simulink model "IM_Global_Control"  (R2021a)
settings: Solver=FixedStepDiscrete  StartTime=0.0  StopTime=10.0  FixedStep=1e-5  RelTol=1e-3
undefined symbols (not defined in the file): DiscIntNeverNeededParam, sigbuilder_block
libraries: simulink x4
settings Model: Creator=Mehra  LastModifiedBy=Mehra

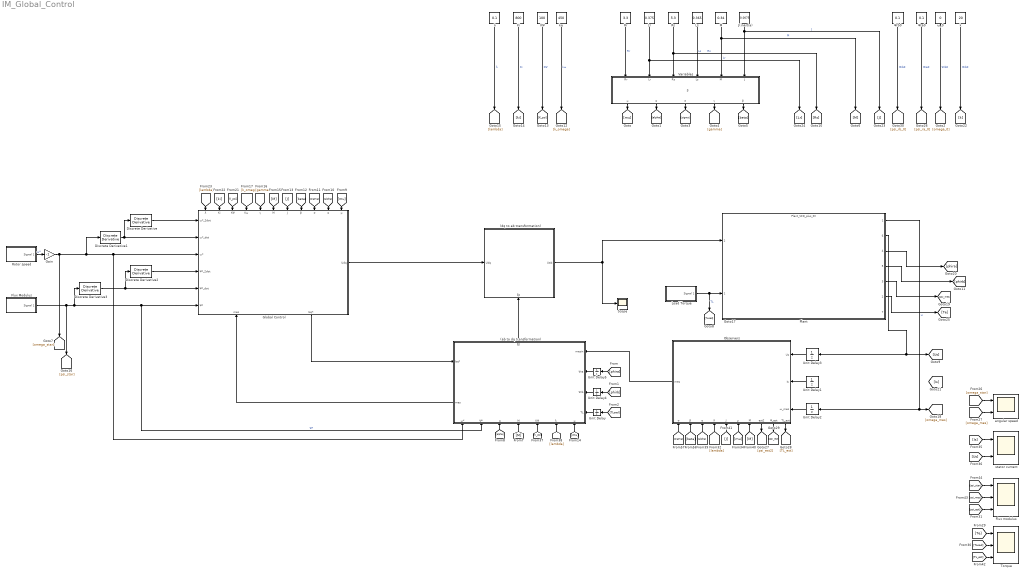
== system IM_Global_Control ==
  note: β
  (ab to dq transformation) : Subsystem
      settings: PortSchema="{\"entries\":[{\"content\":{\"sides\":[{\"content\":{\"connectorIds\":[\"In1\",\"Out2\"]},\"type\":\"ConnectorPlacement.EquallySpacedRectSide\",\"uuid\":\"954ddc6c-32ec-4fca-997a-51b3ced09e6e\"},{\"content\":{\"connectorIds\":[\"In9\",\"In10\",\"In11\",\"In12\"],\"side\":\"RIGHT\"},\"type\":\"ConnectorPlacement.EquallySpacedRectSide\",\"uuid\":\"d23f0106-fd66-41c5-9167-f0bfa2e5f0d7\"},{\"content\":{\"connectorIds\":[\"Out1\"],\"side\":\"TOP\"},\"type\":\"ConnectorPlacement.EquallySpacedRectSide\",\"uuid\":\"ec2ab734-74ce-4c08-89a8-e0d0cab377a3\"},{\"content\":{\"connectorIds\":[\"In2\",\"In3\",\"In4\",\"In5\",\"In6\",\"In7\",\"In8\"],\"side\":\"BOTTOM\"},\"type\":\"ConnectorPlacement.EquallySpacedRectSide\",\"uuid\":\"e8fbabf1-c1e7-4b41-8038-4f25f2d2c141\"}]},\"type\":\"ConnectorPlacement.EquallySpacedConnector\",\"uuid\":\"2eb72d65-4150-4441-ba17-035a64db8a78\"}],\"packageUris\":[\"http://schema.mathworks.com/mf0/Connector/R2020b\"],\"version\":\"1.0\"}"
  (dq to ab transformation) : Subsystem
      settings: PortSchema="{\"entries\":[{\"content\":{\"sides\":[{\"content\":{\"connectorIds\":[\"In1\"]},\"type\":\"ConnectorPlacement.EquallySpacedRectSide\",\"uuid\":\"fcc9e9c0-f3ff-45b3-b4d9-89988d9b9a34\"},{\"content\":{\"connectorIds\":[\"Out1\"],\"side\":\"RIGHT\"},\"type\":\"ConnectorPlacement.EquallySpacedRectSide\",\"uuid\":\"b8117d1c-eda8-48ca-a376-b80f3451eb1b\"},{\"content\":{\"connectorIds\":[],\"side\":\"TOP\"},\"type\":\"ConnectorPlacement.EquallySpacedRectSide\",\"uuid\":\"632a2e27-4ebf-4489-a7a1-4102ed33f7de\"},{\"content\":{\"connectorIds\":[\"In2\"],\"side\":\"BOTTOM\"},\"type\":\"ConnectorPlacement.EquallySpacedRectSide\",\"uuid\":\"b1ed2b98-7899-49a7-98d1-ff7a05505f88\"}]},\"type\":\"ConnectorPlacement.EquallySpacedConnector\",\"uuid\":\"0e689d41-d128-44ad-a484-465e7f7df4f8\"}],\"packageUris\":[\"http://schema.mathworks.com/mf0/Connector/R2020b\"],\"version\":\"1.0\"}"
  Discrete Derivative{,1..3} (4 alike) : simulink/Discrete/Discrete Derivative  gainval=1.0  ICPrevScaledInput=0.0  OutMin=[]  OutMax=[]  OutDataType=fixdt(1, 16)  OutScaling=2^-10  DoSatur=off
  Flux Modulus : Subsystem  Tag=STV Subsys  LoadFcn=sigbuilder_block('load');  StartFcn=sigbuilder_block('start');  StopFcn=sigbuilder_block('stop');  ClipboardFcn=sigbuilder_block('clipboard');  mask(Sigbuilder block){tuvar=[0:10]}
      mask help: Simulink:masks:SigbuilderBlock_MD
      mask init:
      | if ~strcmp(get_param(bdroot(gcbh),'SimulationStatus'),'stopped') tuvar = sigbuilder_block('maskInit'); end
      settings: CopyFcn=sigbuilder_block('copy');  DeleteFcn=sigbuilder_block('delete');  ModelCloseFcn=sigbuilder_block('modelClose');  PreSaveFcn=sigbuilder_block('preSave');  PauseFcn=sigbuilder_block('pause');  ContinueFcn=sigbuilder_block('continue');  NameChangeFcn=sigbuilder_block('namechange');  OpenFcn=sigbuilder_block('open',[433.8 177.6 550.8 400.2 ]);  CloseFcn=sigbuilder_block('close');
      mask Display: plot(0, 0, 100, 100,[2, 2, 32, 32, 2], [68, 8, 8, 68, 68],[32, 2], [38, 38], [32, 19, 2],[53, 60, 44], [32, 17, 17, 2],[16, 16, 31, 31]);txt = getActiveGroup(gcbh);text(2, 100, txt,'verticalAlignment', 'top');
  Flux modulus : Scope  NumInputPorts=3
  Gain : Gain  Gain=-1
  Global Control : Subsystem
      settings: PortSchema="{\"entries\":[{\"content\":{\"sides\":[{\"content\":{\"connectorIds\":[\"In1\",\"In2\",\"In3\",\"In4\",\"In5\",\"In6\"]},\"type\":\"ConnectorPlacement.EquallySpacedRectSide\",\"uuid\":\"d7ac22ed-73dc-4923-8a02-de2b77bc4b56\"},{\"content\":{\"connectorIds\":[\"Out1\"],\"side\":\"RIGHT\"},\"type\":\"ConnectorPlacement.EquallySpacedRectSide\",\"uuid\":\"0ed82d2d-ac01-4440-b414-7b739c3193d9\"},{\"content\":{\"connectorIds\":[\"In7\",\"In8\",\"In9\",\"In10\",\"In11\",\"In12\",\"In13\",\"In14\",\"In15\",\"In16\",\"In17\"],\"side\":\"TOP\"},\"type\":\"ConnectorPlacement.EquallySpacedRectSide\",\"uuid\":\"be3374af-951c-49b1-9762-82694f1e2186\"},{\"content\":{\"connectorIds\":[\"In18\",\"Out2\"],\"side\":\"BOTTOM\"},\"type\":\"ConnectorPlacement.EquallySpacedRectSide\",\"uuid\":\"0e0cdf13-df45-4d83-96ab-036d988b30e8\"}]},\"type\":\"ConnectorPlacement.EquallySpacedConnector\",\"uuid\":\"01640f11-0e41-43e3-9a6d-1e07964cb7e3\"}],\"packageUris\":[\"http://schema.mathworks.com/mf0/Connector/R2020b\"],\"version\":\"1.0\"}"
  J(inertia) : Constant  Value=0.0075
  Ki : Constant  Value=800
  KΨ : Constant  Value=100
  Load Torque : Subsystem  Tag=STV Subsys  LoadFcn=sigbuilder_block('load');  StartFcn=sigbuilder_block('start');  StopFcn=sigbuilder_block('stop');  ClipboardFcn=sigbuilder_block('clipboard');  mask(Sigbuilder block){tuvar=[0:10]}
      mask help: Simulink:masks:SigbuilderBlock_MD
      mask init:
      | if ~strcmp(get_param(bdroot(gcbh),'SimulationStatus'),'stopped') tuvar = sigbuilder_block('maskInit'); end
      settings: CopyFcn=sigbuilder_block('copy');  DeleteFcn=sigbuilder_block('delete');  ModelCloseFcn=sigbuilder_block('modelClose');  PreSaveFcn=sigbuilder_block('preSave');  PauseFcn=sigbuilder_block('pause');  ContinueFcn=sigbuilder_block('continue');  NameChangeFcn=sigbuilder_block('namechange');  OpenFcn=sigbuilder_block('open',[418.2 149.4 550.8 400.2 ]);  CloseFcn=sigbuilder_block('close');
      mask Display: plot(0, 0, 100, 100,[2, 2, 32, 32, 2], [68, 8, 8, 68, 68],[32, 2], [38, 38], [32, 19, 2],[53, 60, 44], [32, 17, 17, 2],[16, 16, 31, 31]);txt = getActiveGroup(gcbh);text(2, 100, txt,'verticalAlignment', 'top');
  Lr : Constant  Value=0.375
  Ls : Constant  Value=0.365
  M : Constant  Value=0.34
  Observers : Subsystem
      settings: PortSchema="{\"entries\":[{\"content\":{\"sides\":[{\"content\":{\"connectorIds\":[\"In1\",\"In2\",\"In3\"]},\"type\":\"ConnectorPlacement.EquallySpacedRectSide\",\"uuid\":\"a75d3ae5-6cbc-4a81-a14c-a9660c01f407\"},{\"content\":{\"connectorIds\":[\"Out1\"],\"side\":\"RIGHT\"},\"type\":\"ConnectorPlacement.EquallySpacedRectSide\",\"uuid\":\"810d57cb-fd51-4174-8429-89dcdd7ccf2e\"},{\"content\":{\"connectorIds\":[],\"side\":\"TOP\"},\"type\":\"ConnectorPlacement.EquallySpacedRectSide\",\"uuid\":\"084f081f-5dfb-4a02-b6e7-31480db1dce2\"},{\"content\":{\"connectorIds\":[\"Out2\",\"Out3\",\"Out4\",\"In4\",\"In5\",\"In6\",\"In7\",\"In8\",\"In9\",\"In10\"],\"side\":\"BOTTOM\"},\"type\":\"ConnectorPlacement.EquallySpacedRectSide\",\"uuid\":\"ad0ec213-e44f-4285-8d86-85a591b1b38d\"}]},\"type\":\"ConnectorPlacement.EquallySpacedConnector\",\"uuid\":\"2b9d98d5-99d7-45ac-aedf-db0f18522aa3\"}],\"packageUris\":[\"http://schema.mathworks.com/mf0/Connector/R2020b\"],\"version\":\"1.0\"}"
  Plant : ModelReference  ModelNameDialog=Plant_VFD_plus_IM.slx  SimulationMode=Normal  ModelReferenceVersion=1.1162
      settings: PortSchema="{\"entries\":[{\"content\":{\"sides\":[{\"content\":{\"connectorIds\":[\"In2\",\"In1\"]},\"type\":\"ConnectorPlacement.EquallySpacedRectSide\",\"uuid\":\"ada58a5e-1472-4b56-9b66-b9d99a7685f5\"},{\"content\":{\"connectorIds\":[\"Out1\",\"Out6\",\"Out4\",\"Out5\",\"Out3\",\"Out2\",\"Out7\"],\"side\":\"RIGHT\"},\"type\":\"ConnectorPlacement.EquallySpacedRectSide\",\"uuid\":\"42b90cbf-75bc-499b-a3c1-3c9b222f35d5\"},{\"content\":{\"connectorIds\":[],\"side\":\"TOP\"},\"type\":\"ConnectorPlacement.EquallySpacedRectSide\",\"uuid\":\"c9789acb-3ca3-4ea3-b872-57f6132d0fb2\"},{\"content\":{\"connectorIds\":[],\"side\":\"BOTTOM\"},\"type\":\"ConnectorPlacement.EquallySpacedRectSide\",\"uuid\":\"000e5c64-e399-41cd-9c94-e7f3b3194d1a\"}]},\"type\":\"ConnectorPlacement.EquallySpacedConnector\",\"uuid\":\"64f9ad12-90f4-47a3-8034-21f20e745ad8\"}],\"packageUris\":[\"http://schema.mathworks.com/mf0/Connector/R2020b\"],\"version\":\"1.0\"}"
  Rotor speed : Subsystem  Tag=STV Subsys  LoadFcn=sigbuilder_block('load');  StartFcn=sigbuilder_block('start');  StopFcn=sigbuilder_block('stop');  ClipboardFcn=sigbuilder_block('clipboard');  mask(Sigbuilder block){tuvar=[0:10]}
      mask help: Simulink:masks:SigbuilderBlock_MD
      mask init:
      | if ~strcmp(get_param(bdroot(gcbh),'SimulationStatus'),'stopped') tuvar = sigbuilder_block('maskInit'); end
      settings: CopyFcn=sigbuilder_block('copy');  DeleteFcn=sigbuilder_block('delete');  ModelCloseFcn=sigbuilder_block('modelClose');  PreSaveFcn=sigbuilder_block('preSave');  PauseFcn=sigbuilder_block('pause');  ContinueFcn=sigbuilder_block('continue');  NameChangeFcn=sigbuilder_block('namechange');  OpenFcn=sigbuilder_block('open',[418.2 149.4 550.8 400.2 ]);  CloseFcn=sigbuilder_block('close');
      mask Display: plot(0, 0, 100, 100,[2, 2, 32, 32, 2], [68, 8, 8, 68, 68],[32, 2], [38, 38], [32, 19, 2],[53, 60, 44], [32, 17, 17, 2],[16, 16, 31, 31]);txt = getActiveGroup(gcbh);text(2, 100, txt,'verticalAlignment', 'top');
  Rr : Constant  Value=3.3
  Rs : Constant  Value=5.3
  Scope : Scope
  Torque : Scope  NumInputPorts=3
  Unit Delay{,1..5} (6 alike) : UnitDelay  SampleTime=-1  HasFrameUpgradeWarning=on
  Variables : Subsystem
  angular speed : Scope  NumInputPorts=2
  k : Constant  Value=20
  kω : Constant  Value=450
  stator current : Scope  NumInputPorts=2
  Ψra0 : Constant  Value=0.1
  Ψrb0 : Constant  Value=0.1
  λ : Constant  Value=0.1
  ω_0 : Constant  Value=0
  wires:
  [sigma] -> Global Control/15(σ)
  [Us] -> stator current/2
  [omega_star] -> angular speed/1
  [ki] -> Global Control/8(Ki)
  [K_psi] -> Global Control/9(KΨ)
  [omega_mes] -> angular speed/2
  Discrete Derivative3/1 -> Discrete Derivative2/1, Global Control/5(Ψ*_dot)
  [alpha] -> (ab to dq transformation)/4(α)
  [lambda] -> Global Control/7(λ)
  [k_omega] -> Global Control/10(Kω)
  Discrete Derivative/1 -> Global Control/1(ω*_2dot)
  [M] -> (ab to dq transformation)/5(M)
  [psi_star] -> Flux modulus/1
  [TLoad] -> Torque/2
  [M] -> Global Control/12(M)
  Observers/3(Ψ_est) -> [psi_est]
  [Te] -> Torque/1
  [Is] -> stator current/1
  [TL_est] -> Torque/3
  Unit Delay2/1 -> Observers/3(ω_mes)
  (ab to dq transformation)/1(ξ0) -> (dq to ab transformation)/2(ξ0)
  Observers/1(mes) -> (ab to dq transformation)/9(mesin)
  Flux Modulus/1(Signal 1) -> Discrete Derivative3/1, Global Control/6(Ψ*), (ab to dq transformation)/3(Ψ*), [psi_star]  "Ψ*"
  Observers/4(est2) -> [psi_est2]
  Discrete Derivative1/1 -> Discrete Derivative/1, Global Control/2(ω*_dot)
  [mu] -> Global Control/17(µ)
  [beta] -> Global Control/14(β)
  (dq to ab transformation)/1(Uab) -> Scope/1, Plant/2
  [sigma] -> Observers/10(σ)
  [beta] -> Observers/9(β)
  [M] -> Observers/4(M)
  [alpha] -> Observers/8(α)
  [lambda] -> Observers/7(λ)
  [psi_est] -> Flux modulus/3
  Observers/2(TL_est) -> [TL_est]
  [mu] -> Observers/5(µ)
  Global Control/1(Udq) -> (dq to ab transformation)/1(Udq)
  [J] -> Global Control/13(J)
  [gamma] -> Global Control/11(γ)
  [alpha] -> Global Control/16(α)
  [K_psi] -> (ab to dq transformation)/6(KΨ)
  (ab to dq transformation)/2(mes) -> Global Control/18(mes)
  Global Control/2(Isq*) -> (ab to dq transformation)/1(Isq*)
  Discrete Derivative2/1 -> Global Control/4(Ψ*_2dot)
  Rotor speed/1(Signal 1) -> Gain/1  "ω*"
  [lambda] -> (ab to dq transformation)/7(λ)
  [mu] -> (ab to dq transformation)/8(µ)
  [J] -> Observers/6(J)
  [psi_mes] -> Flux modulus/2
  Plant/2 -> [Te]
  Load Torque/1(Signal 1) -> [TLoad], Plant/1  "TL"
  Plant/3 -> [psi_mes]
  Plant/1 -> [omega_mes], Unit Delay2/1  "ω"
  ? -> [Is], Unit Delay1/1
  Plant/6 -> Unit Delay3/1, [Us]
  Unit Delay1/1 -> Observers/2(Is)
  Unit Delay3/1 -> Observers/1(Us)
  Gain/1 -> Discrete Derivative1/1, Global Control/3(ω*), (ab to dq transformation)/2(ω*), [omega_star]
  Plant/5 -> [phirb]
  Plant/4 -> [phira]
  [phira] -> Unit Delay5/1
  [phirb] -> Unit Delay4/1
  [TLoad] -> Unit Delay/1
  Unit Delay/1 -> (ab to dq transformation)/12(TL)
  Unit Delay4/1 -> (ab to dq transformation)/11(Ψrb)
  Unit Delay5/1 -> (ab to dq transformation)/10(Ψra)
  Variables/3(σ) -> [sigma]
  k/1 -> [k]  "Ψrb0"
  Rs/1 -> [Rs], Variables/3(Rs)  "Rs"
  M/1 -> [M], Variables/5(M)  "M"
  Ψrb0/1 -> [psi_rb_0]  "Ψrb0"
  Variables/4(γ) -> [gamma]
  Ψra0/1 -> [psi_ra_0]  "Ψra0"
  Ls/1 -> Variables/4(Ls)  "Ls"
  Variables/2(α) -> [alpha]
  Rr/1 -> Variables/1(Rr)  "Rr"
  ω_0/1 -> [omega_0]  "Ψrb0"
  Variables/5(β) -> [beta]
  Lr/1 -> [Lr], Variables/2(Lr)  "Lr"
  Variables/1(µ) -> [mu]
  J(inertia)/1 -> [J], Variables/6(J)  "J"
  KΨ/1 -> [K_psi]  "KΨ"
  λ/1 -> [lambda]  "λ"
  Ki/1 -> [ki]  "Ki"
  kω/1 -> [k_omega]  "kω"

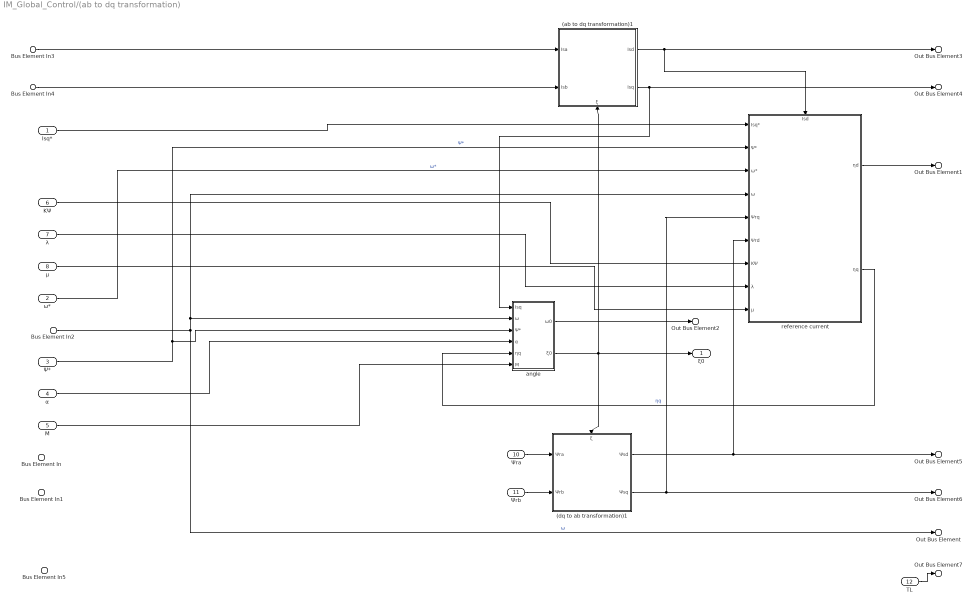
== system IM_Global_Control/(ab to dq transformation) ==
  Isq* : Inport
  ω* : Inport  Port=2
  Ψ* : Inport  Port=3
  α : Inport  Port=4
  M : Inport  Port=5
  KΨ : Inport  Port=6
  λ : Inport  Port=7
  µ : Inport  Port=8
  Bus Element In4 : Inport  Port=9  PortName=mesin  Element=Isb
  Bus Element In : Inport  Port=9  PortName=mesin  Element=Ψra
  Bus Element In1 : Inport  Port=9  PortName=mesin  Element=Ψrb
  Bus Element In2 : Inport  Port=9  PortName=mesin  Element=ω
  Bus Element In3 : Inport  Port=9  PortName=mesin  Element=Isa
  Bus Element In5 : Inport  Port=9  PortName=mesin  Element=TL
  Ψra : Inport  Port=10
  Ψrb : Inport  Port=11
  TL : Inport  Port=12
  (ab to dq transformation)1 : Subsystem
      settings: PortSchema="{\"entries\":[{\"content\":{\"sides\":[{\"content\":{\"connectorIds\":[\"In1\",\"In2\"]},\"type\":\"ConnectorPlacement.EquallySpacedRectSide\",\"uuid\":\"5c330d99-0e0d-44c6-96f8-2a2206da92f9\"},{\"content\":{\"connectorIds\":[\"Out1\",\"Out2\"],\"side\":\"RIGHT\"},\"type\":\"ConnectorPlacement.EquallySpacedRectSide\",\"uuid\":\"d01d6d1d-3c02-43a0-8f85-93fe8d575b38\"},{\"content\":{\"connectorIds\":[],\"side\":\"TOP\"},\"type\":\"ConnectorPlacement.EquallySpacedRectSide\",\"uuid\":\"e1acbeec-a08c-47b9-8afb-d107cbf7174f\"},{\"content\":{\"connectorIds\":[\"In3\"],\"side\":\"BOTTOM\"},\"type\":\"ConnectorPlacement.EquallySpacedRectSide\",\"uuid\":\"e8043408-ca76-4c99-9608-24b05f44ef39\"}]},\"type\":\"ConnectorPlacement.EquallySpacedConnector\",\"uuid\":\"9536c8a8-a5cc-4817-9165-61d2eb9b262d\"}],\"packageUris\":[\"http://schema.mathworks.com/mf0/Connector/R2020b\"],\"version\":\"1.0\"}"
  (dq to ab transformation)1 : Subsystem
      settings: PortSchema="{\"entries\":[{\"content\":{\"sides\":[{\"content\":{\"connectorIds\":[\"In1\",\"In2\"]},\"type\":\"ConnectorPlacement.EquallySpacedRectSide\",\"uuid\":\"5c330d99-0e0d-44c6-96f8-2a2206da92f9\"},{\"content\":{\"connectorIds\":[\"Out1\",\"Out2\"],\"side\":\"RIGHT\"},\"type\":\"ConnectorPlacement.EquallySpacedRectSide\",\"uuid\":\"d01d6d1d-3c02-43a0-8f85-93fe8d575b38\"},{\"content\":{\"connectorIds\":[\"In3\"],\"side\":\"TOP\"},\"type\":\"ConnectorPlacement.EquallySpacedRectSide\",\"uuid\":\"e1acbeec-a08c-47b9-8afb-d107cbf7174f\"},{\"content\":{\"connectorIds\":[],\"side\":\"BOTTOM\"},\"type\":\"ConnectorPlacement.EquallySpacedRectSide\",\"uuid\":\"e8043408-ca76-4c99-9608-24b05f44ef39\"}]},\"type\":\"ConnectorPlacement.EquallySpacedConnector\",\"uuid\":\"9536c8a8-a5cc-4817-9165-61d2eb9b262d\"}],\"packageUris\":[\"http://schema.mathworks.com/mf0/Connector/R2020b\"],\"version\":\"1.0\"}"
  angle : Subsystem
  reference current : Subsystem
      settings: PortSchema="{\"entries\":[{\"content\":{\"sides\":[{\"content\":{\"connectorIds\":[\"In1\",\"In2\",\"In3\",\"In4\",\"In5\",\"In6\",\"In7\",\"In8\",\"In9\"]},\"type\":\"ConnectorPlacement.EquallySpacedRectSide\",\"uuid\":\"20835a9a-3790-4a84-a1cf-3b356ea8ce55\"},{\"content\":{\"connectorIds\":[\"Out1\",\"Out2\"],\"side\":\"RIGHT\"},\"type\":\"ConnectorPlacement.EquallySpacedRectSide\",\"uuid\":\"c7be742b-d8ac-4ccc-8e57-82e64648b197\"},{\"content\":{\"connectorIds\":[\"In10\"],\"side\":\"TOP\"},\"type\":\"ConnectorPlacement.EquallySpacedRectSide\",\"uuid\":\"50541cb9-7339-4b7f-ab09-a0a36464c354\"}]},\"type\":\"ConnectorPlacement.EquallySpacedConnector\",\"uuid\":\"b3e3bb9d-f2d1-405f-a9ca-c5a471d81e39\"}],\"packageUris\":[\"http://schema.mathworks.com/mf0/Connector/R2020b\"],\"version\":\"1.0\"}"
  ξ0 : Outport
  Out Bus Element : Outport  Port=2  PortName=mes  Element=ω
  Out Bus Element1 : Outport  Port=2  PortName=mes  Element=ηd
  Out Bus Element2 : Outport  Port=2  PortName=mes  Element=ω0
  Out Bus Element3 : Outport  Port=2  PortName=mes  Element=Isd
  Out Bus Element4 : Outport  Port=2  PortName=mes  Element=Isq
  Out Bus Element5 : Outport  Port=2  PortName=mes  Element=Ψrd
  Out Bus Element6 : Outport  Port=2  PortName=mes  Element=Ψrq
  Out Bus Element7 : Outport  Port=2  PortName=mes  Element=TL
  wires:
  Ψ*/1 -> angle/3(Ψ*), reference current/2(Ψ*)  "Ψ*"
  Bus Element In2/1 -> Out Bus Element/1, angle/2(ω), reference current/4(ω)  "ω"
  Bus Element In3/1 -> (ab to dq transformation)1/1(Isa)
  Bus Element In4/1 -> (ab to dq transformation)1/2(Isb)
  reference current/2(ηq) -> angle/5(ηq)  "ηq"
  Isq*/1 -> reference current/1(Isq*)
  ω*/1 -> reference current/3(ω*)  "ω*"
  µ/1 -> reference current/9(µ)
  λ/1 -> reference current/8(λ)
  KΨ/1 -> reference current/7(KΨ)
  reference current/1(ηd) -> Out Bus Element1/1
  (ab to dq transformation)1/1(Isd) -> Out Bus Element3/1, reference current/10(Isd)
  (dq to ab transformation)1/1(Ψsd) -> Out Bus Element5/1, reference current/6(Ψrd)
  (dq to ab transformation)1/2(Ψsq) -> Out Bus Element6/1, reference current/5(Ψrq)
  angle/2(ξ0) -> ξ0/1, (dq to ab transformation)1/3(ξ), (ab to dq transformation)1/3(ξ)
  (ab to dq transformation)1/2(Isq) -> angle/1(Isq), Out Bus Element4/1
  α/1 -> angle/4(α)
  M/1 -> angle/6(M)
  angle/1(ω0) -> Out Bus Element2/1
  Ψra/1 -> (dq to ab transformation)1/1(Ψra)
  Ψrb/1 -> (dq to ab transformation)1/2(Ψrb)
  TL/1 -> Out Bus Element7/1

== system IM_Global_Control/(dq to ab transformation) ==
  In Bus Element : Inport  PortName=Udq  Element=usd
  In Bus Element1 : Inport  PortName=Udq  Element=usq
  ξ0 : Inport  Port=2
  Cos : Trigonometry  Operator=cos
  Cos1 : Trigonometry
  Product{,1..3} (4 alike) : Product
  Sin : Trigonometry
  Sin1 : Trigonometry  Operator=cos
  Subtract : Sum  Inputs=+-
  Subtract1 : Sum
  Out Bus Element : Outport  PortName=Uab  Element=Usa
  Out Bus Element1 : Outport  PortName=Uab  Element=Usb
  wires:
  Subtract1/1 -> Out Bus Element1/1  "Usb"
  Subtract/1 -> Out Bus Element/1  "Usa"
  ξ0/1 -> Sin1/1, Cos1/1, Sin/1, Cos/1  "ξ0"
  Cos/1 -> Product/1
  Sin/1 -> Product1/2
  Cos1/1 -> Product2/1
  Sin1/1 -> Product3/2
  In Bus Element/1 -> Product2/2, Product/2  "usd"
  In Bus Element1/1 -> Product3/1, Product1/1  "usq"
  Product/1 -> Subtract/1
  Product1/1 -> Subtract/2
  Product2/1 -> Subtract1/1
  Product3/1 -> Subtract1/2

== system IM_Global_Control/Flux Modulus ==
  Demux : Demux  Tag=STV Demux  Outputs=1
      settings: DisplayOption=none
  FromWs : FromWorkspace  Tag=STV FromWs  VariableName=tuvar
      SigBuilderData=|
      | common.afterFinalStr = 'Extrapolate'
      | common.sampleTime = 0
      | dataSet.timeRange = [0 10]
      | dataSet.name = 'Group 1'
      | sbobj.Groups.Name = 'Group 1'
      | sbobj.Groups.Signals.Name = 'Signal 1'
      | sbobj.Groups.Signals.XData = [0 0.32 1.5 1.8 10]
      | sbobj.Groups.Signals.YData = [0.001 1.16 1.16 0.5 0.5]
  Signal 1 : Outport  Tag=STV Outport
  wires:
  Demux/1 -> Signal 1/1
  FromWs/1 -> Demux/1

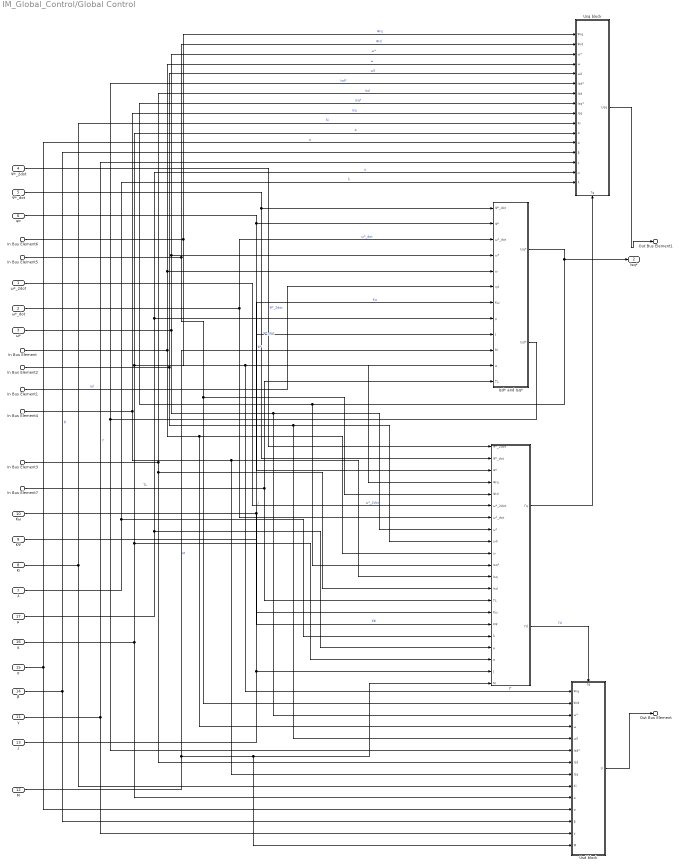
== system IM_Global_Control/Global Control ==
  ω*_2dot : Inport
  ω*_dot : Inport  Port=2
  ω* : Inport  Port=3
  Ψ*_2dot : Inport  Port=4
  Ψ*_dot : Inport  Port=5
  Ψ* : Inport  Port=6
  λ : Inport  Port=7
  Ki : Inport  Port=8
  KΨ : Inport  Port=9
  Kω : Inport  Port=10
  γ : Inport  Port=11
  M : Inport  Port=12
  J : Inport  Port=13
  β : Inport  Port=14
  σ : Inport  Port=15
  α : Inport  Port=16
  µ : Inport  Port=17
  In Bus Element : Inport  Port=18  PortName=mes  Element=ω
  In Bus Element1 : Inport  Port=18  PortName=mes  Element=ηd
  In Bus Element2 : Inport  Port=18  PortName=mes  Element=ω0
  In Bus Element3 : Inport  Port=18  PortName=mes  Element=Isd
  In Bus Element4 : Inport  Port=18  PortName=mes  Element=Isq
  In Bus Element5 : Inport  Port=18  PortName=mes  Element=Ψrd
  In Bus Element6 : Inport  Port=18  PortName=mes  Element=Ψrq
  In Bus Element7 : Inport  Port=18  PortName=mes  Element=TL
  Isd* and Isq* : Subsystem
  Usd block : Subsystem
      settings: PortSchema="{\"entries\":[{\"content\":{\"sides\":[{\"content\":{\"connectorIds\":[\"In1\",\"In2\",\"In3\",\"In4\",\"In5\",\"In6\",\"In7\",\"In8\",\"In9\",\"In10\",\"In11\",\"In12\",\"In13\",\"In14\"]},\"type\":\"ConnectorPlacement.EquallySpacedRectSide\",\"uuid\":\"0b3b8e54-774f-4e59-b7ae-fc3f76f7169f\"},{\"content\":{\"connectorIds\":[\"Out1\"],\"side\":\"RIGHT\"},\"type\":\"ConnectorPlacement.EquallySpacedRectSide\",\"uuid\":\"160f327c-323c-4922-a7f8-789847ab983f\"},{\"content\":{\"connectorIds\":[\"In15\"],\"side\":\"TOP\"},\"type\":\"ConnectorPlacement.EquallySpacedRectSide\",\"uuid\":\"f6ec24e2-9a41-47bb-ba15-6aba8409f45e\"}]},\"type\":\"ConnectorPlacement.EquallySpacedConnector\",\"uuid\":\"52a2cf74-17c5-48e5-8a86-53458a7f2c84\"}],\"packageUris\":[\"http://schema.mathworks.com/mf0/Connector/R2020b\"],\"version\":\"1.0\"}"
  Usq block : Subsystem
      settings: PortSchema="{\"entries\":[{\"content\":{\"sides\":[{\"content\":{\"connectorIds\":[\"In1\",\"In2\",\"In3\",\"In4\",\"In5\",\"In6\",\"In7\",\"In8\",\"In9\",\"In10\",\"In11\",\"In12\",\"In13\",\"In14\",\"In15\",\"In16\"]},\"type\":\"ConnectorPlacement.EquallySpacedRectSide\",\"uuid\":\"e0829cb0-14ba-4968-8b37-82965b41b0aa\"},{\"content\":{\"connectorIds\":[\"Out1\"],\"side\":\"RIGHT\"},\"type\":\"ConnectorPlacement.EquallySpacedRectSide\",\"uuid\":\"1d4d172a-7610-496b-b8fe-18e12381e6b4\"},{\"content\":{\"connectorIds\":[],\"side\":\"TOP\"},\"type\":\"ConnectorPlacement.EquallySpacedRectSide\",\"uuid\":\"0fc98001-c07f-432d-975f-c7605f9f4273\"},{\"content\":{\"connectorIds\":[\"In17\"],\"side\":\"BOTTOM\"},\"type\":\"ConnectorPlacement.EquallySpacedRectSide\",\"uuid\":\"89865e84-6121-4a9b-9592-d6a2eae0e50b\"}]},\"type\":\"ConnectorPlacement.EquallySpacedConnector\",\"uuid\":\"d7e7f672-cce9-4dd7-86e0-c30144b95288\"}],\"packageUris\":[\"http://schema.mathworks.com/mf0/Connector/R2020b\"],\"version\":\"1.0\"}"
  Γ : Subsystem
  Out Bus Element : Outport  PortName=Udq  Element=usd
  Out Bus Element1 : Outport  PortName=Udq  Element=usq
  Isq* : Outport  Port=2
  wires:
  Ψ*_2dot/1 -> Γ/1(Ψ*_2dot)  "Ψ*_2dot"
  Ψ*_dot/1 -> Isd* and Isq*/1(Ψ*_dot), Γ/2(Ψ*_dot)  "Ψ*_dot"
  Ψ*/1 -> Isd* and Isq*/2(Ψ*), Γ/3(Ψ*)  "Ψ*"
  In Bus Element6/1 -> Usq block/1(Ψrq), Γ/4(Ψrq), Usd block/1(Ψrq)  "Ψrq"
  In Bus Element5/1 -> Usq block/2(Ψrd), Γ/5(Ψrd), Usd block/2(Ψrd)  "Ψrd"
  ω*_2dot/1 -> Γ/6(ω*_2dot)  "ω*_2dot"
  ω*_dot/1 -> Isd* and Isq*/3(ω*_dot), Γ/7(ω*_dot)  "ω*_dot"
  ω*/1 -> Usd block/3(ω*), Γ/8(ω*), Isd* and Isq*/4(ω*), Usq block/3(ω*)  "ω*"
  In Bus Element2/1 -> Usq block/5(ω0), Usd block/5(ω0), Γ/9(ω0)  "ω0"
  In Bus Element/1 -> Usd block/4(ω), Γ/10(ω), Isd* and Isq*/5(ω), Usq block/4(ω)  "ω"
  Isd* and Isq*/1(Isq*) -> Isq*/1, Usq block/8(Isq*), Γ/11(Isq*)  "Isq*"
  In Bus Element4/1 -> Usq block/9(Isq), Γ/12(Isq), Usd block/8(Isq)  "Isq"
  In Bus Element3/1 -> Usq block/7(Isd), Γ/13(Isd), Usd block/7(Isd)  "Isd"
  In Bus Element7/1 -> Isd* and Isq*/12(TL), Γ/14(TL)  "TL"
  Kω/1 -> Γ/15(Kω), Isd* and Isq*/7(Kω)  "Kω"
  KΨ/1 -> Γ/16(KΨ)  "KΨ"
  λ/1 -> Γ/17(λ), Usq block/16(λ)  "λ"
  µ/1 -> Isd* and Isq*/8(µ), Usq block/15(µ), Γ/18(µ)  "µ"
  α/1 -> Γ/19(α), Usq block/11(α), Isd* and Isq*/11(α), Usd block/10(α)  "α"
  J/1 -> Γ/20(J), Isd* and Isq*/9(J)  "J"
  M/1 -> Isd* and Isq*/10(M), Γ/21(M), Usd block/14(M)  "M"
  Isd* and Isq*/2(Isd*) -> Usd block/6(Isd*), Usq block/6(Isd*)  "Isd*"
  Γ/2(Γd) -> Usd block/15(Γd)  "Γd"
  Ki/1 -> Usq block/10(Ki), Usd block/9(Ki)  "Ki"
  σ/1 -> Usq block/12(σ), Usd block/11(σ)  "σ"
  β/1 -> Usq block/13(β), Usd block/12(β)  "β"
  γ/1 -> Usq block/14(γ), Usd block/13(γ)  "γ"
  Usd block/1(U) -> Out Bus Element/1
  Γ/1(Γq) -> Usq block/17(Γq)
  Usq block/1(Usq) -> Out Bus Element1/1
  In Bus Element1/1 -> Isd* and Isq*/6(ηd)  "ηd"

== system IM_Global_Control/Load Torque ==
  Demux : Demux  Tag=STV Demux  Outputs=1
      settings: DisplayOption=none
  FromWs : FromWorkspace  Tag=STV FromWs  VariableName=tuvar
      SigBuilderData=|
      | common.afterFinalStr = 'Extrapolate'
      | common.sampleTime = 0
      | dataSet.timeRange = [0 10]
      | dataSet.name = 'Group 1'
      | sbobj.Groups.Name = 'Group 1'
      | sbobj.Groups.Signals.Name = 'Signal 1'
      | sbobj.Groups.Signals.XData = [0 0.32 0.32 1 1 10]
      | sbobj.Groups.Signals.YData = [0 0 5.8 5.8 1.8 1.8]
  Signal 1 : Outport  Tag=STV Outport
  wires:
  Demux/1 -> Signal 1/1
  FromWs/1 -> Demux/1

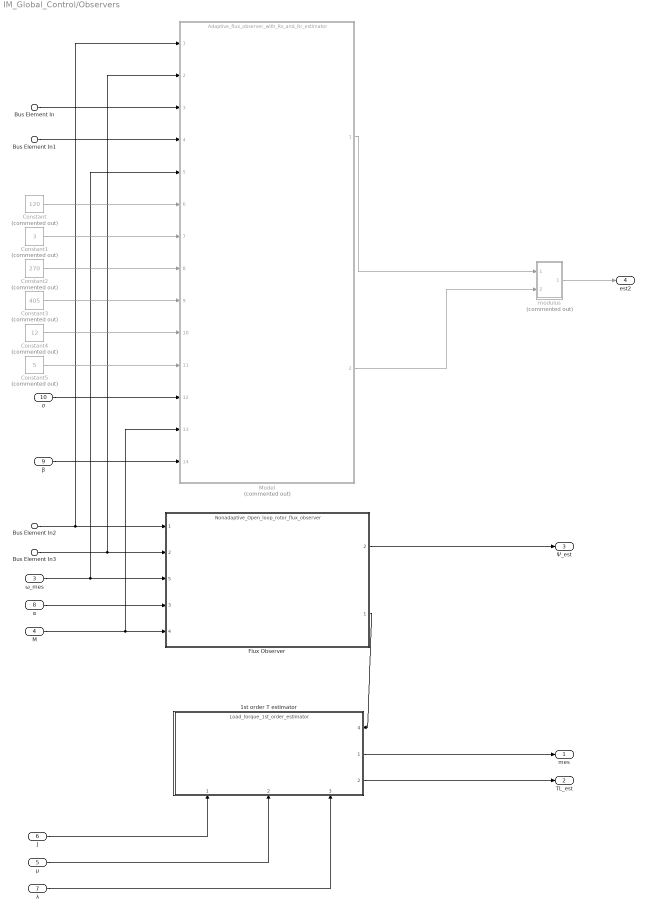
== system IM_Global_Control/Observers ==
  Bus Element In : Inport  PortName=Us  Element=Usa
  Bus Element In1 : Inport  PortName=Us  Element=Usb
  Bus Element In2 : Inport  Port=2  PortName=Is  Element=Isa
  Bus Element In3 : Inport  Port=2  PortName=Is  Element=Isb
  ω_mes : Inport  Port=3
  M : Inport  Port=4
  µ : Inport  Port=5
  J : Inport  Port=6
  λ : Inport  Port=7
  α : Inport  Port=8
  β : Inport  Port=9
  σ : Inport  Port=10
  1st order T estimator : ModelReference  ModelNameDialog=Load_torque_1st_order_estimator.slx  SimulationMode=Normal  ModelReferenceVersion=1.27
      settings: PortSchema="{\"entries\":[{\"content\":{\"sides\":[{\"content\":{\"connectorIds\":[]},\"type\":\"ConnectorPlacement.EquallySpacedRectSide\",\"uuid\":\"cec251cb-6b4e-4904-a832-c5acce82a070\"},{\"content\":{\"connectorIds\":[\"In4\",\"Out1\",\"Out2\"],\"side\":\"RIGHT\"},\"type\":\"ConnectorPlacement.EquallySpacedRectSide\",\"uuid\":\"735376b5-2ddd-4bd3-962c-0ec3161c2740\"},{\"content\":{\"connectorIds\":[],\"side\":\"TOP\"},\"type\":\"ConnectorPlacement.EquallySpacedRectSide\",\"uuid\":\"64a3f3a5-dee8-4d60-ac03-c9c941997ec4\"},{\"content\":{\"connectorIds\":[\"In1\",\"In2\",\"In3\"],\"side\":\"BOTTOM\"},\"type\":\"ConnectorPlacement.EquallySpacedRectSide\",\"uuid\":\"a9b1d046-d6bc-45e1-a3f0-76ce350da922\"}]},\"type\":\"ConnectorPlacement.EquallySpacedConnector\",\"uuid\":\"7512dbd3-06b9-47bd-8f2d-91bb52696950\"}],\"packageUris\":[\"http://schema.mathworks.com/mf0/Connector/R2020b\"],\"version\":\"1.0\"}"
  Constant : Constant  Commented=on  Value=120
  Constant1 : Constant  Commented=on  Value=3
  Constant2 : Constant  Commented=on  Value=270
  Constant3 : Constant  Commented=on  Value=405
  Constant4 : Constant  Commented=on  Value=12
  Constant5 : Constant  Commented=on  Value=5
  Flux Observer : ModelReference  ModelNameDialog=Nonadaptive_Open_loop_rotor_flux_observer  SimulationMode=Normal  ModelReferenceVersion=1.37
      settings: PortSchema="{\"entries\":[{\"content\":{\"sides\":[{\"content\":{\"connectorIds\":[\"In1\",\"In2\",\"In5\",\"In3\",\"In4\"]},\"type\":\"ConnectorPlacement.EquallySpacedRectSide\",\"uuid\":\"57c66cae-f60c-4fa2-8fd5-f5b68222e0bb\"},{\"content\":{\"connectorIds\":[\"Out2\",\"Out1\"],\"side\":\"RIGHT\"},\"type\":\"ConnectorPlacement.EquallySpacedRectSide\",\"uuid\":\"591ff962-71a1-4adf-845c-7b897bc73935\"},{\"content\":{\"connectorIds\":[],\"side\":\"TOP\"},\"type\":\"ConnectorPlacement.EquallySpacedRectSide\",\"uuid\":\"d0e2f489-3eb5-488c-a0b4-9296b4be860b\"}]},\"type\":\"ConnectorPlacement.EquallySpacedConnector\",\"uuid\":\"15b17a83-f5fe-4267-a8df-d0f0282de86a\"}],\"packageUris\":[\"http://schema.mathworks.com/mf0/Connector/R2020b\"],\"version\":\"1.0\"}"
  Model : ModelReference  Commented=on  ModelNameDialog=Adaptive_flux_observer_with_Rs_and_Rr_estimator.slx  SimulationMode=Normal  ModelReferenceVersion=1.223
  modulus : Subsystem  Commented=on
  mes : Outport
  TL_est : Outport  Port=2
  Ψ_est : Outport  Port=3
  est2 : Outport  Port=4
  wires:
  ω_mes/1 -> Model/5, Flux Observer/5
  J/1 -> 1st order T estimator/1
  Flux Observer/1 -> 1st order T estimator/4
  Bus Element In3/1 -> Model/2, Flux Observer/2
  α/1 -> Flux Observer/3
  Bus Element In2/1 -> Model/1, Flux Observer/1
  M/1 -> Model/13, Flux Observer/4
  λ/1 -> 1st order T estimator/3
  µ/1 -> 1st order T estimator/2
  1st order T estimator/1 -> mes/1
  Flux Observer/2 -> Ψ_est/1
  1st order T estimator/2 -> TL_est/1
  β/1 -> Model/14
  σ/1 -> Model/12
  Bus Element In/1 -> Model/3
  Bus Element In1/1 -> Model/4
  Constant/1 -> Model/6
  Constant1/1 -> Model/7
  Constant2/1 -> Model/8
  Constant3/1 -> Model/9
  Constant4/1 -> Model/10
  Constant5/1 -> Model/11
  Model/1 -> modulus/1(1)
  Model/2 -> modulus/2(In2)
  modulus/1(Output) -> est2/1

== system IM_Global_Control/Rotor speed ==
  Demux : Demux  Tag=STV Demux  Outputs=1
      settings: DisplayOption=none
  FromWs : FromWorkspace  Tag=STV FromWs  VariableName=tuvar
      SigBuilderData=|
      | common.afterFinalStr = 'Extrapolate'
      | common.sampleTime = 0
      | dataSet.timeRange = [0 10]
      | dataSet.name = 'Group 1'
      | sbobj.Groups.Name = 'Group 1'
      | sbobj.Groups.Signals.Name = 'Signal 1'
      | sbobj.Groups.Signals.XData = [0 0.32 1 1.5 2 10]
      | sbobj.Groups.Signals.YData = [0 0 100 100 200 200]
  Signal 1 : Outport  Tag=STV Outport
  wires:
  Demux/1 -> Signal 1/1
  FromWs/1 -> Demux/1

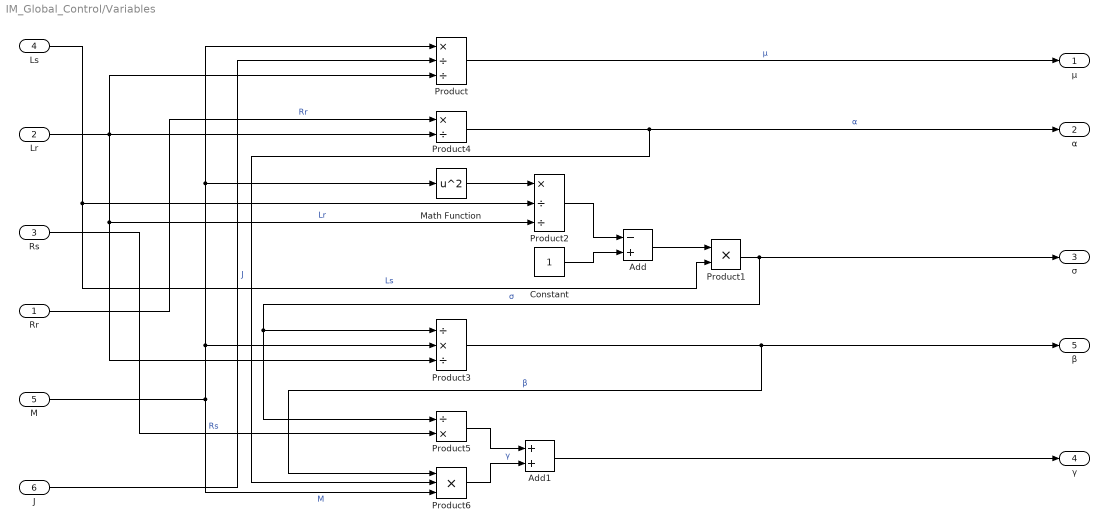
== system IM_Global_Control/Variables ==
  Rr : Inport
  Lr : Inport  Port=2
  Rs : Inport  Port=3
  Ls : Inport  Port=4
  M : Inport  Port=5
  J : Inport  Port=6
  Add : Sum  Inputs=-+
  Add1 : Sum
  Constant : Constant
  Math Function : Math  Operator=square  SaturateOnIntegerOverflow=on
  Product : Product  Inputs=*//
  Product1 : Product
  Product2 : Product  Inputs=*//
  Product3 : Product  Inputs=/*/
  Product4 : Product  Inputs=*/
  Product5 : Product  Inputs=/*
  Product6 : Product  Inputs=3
  µ : Outport
  α : Outport  Port=2
  σ : Outport  Port=3
  γ : Outport  Port=4
  β : Outport  Port=5
  wires:
  M/1 -> Product3/2, Math Function/1, Product/1, Product6/3  "M"
  J/1 -> Product/2  "J"
  Lr/1 -> Product4/2, Product/3, Product2/3, Product3/3  "Lr"
  Product/1 -> µ/1  "µ"
  Add/1 -> Product1/1
  Ls/1 -> Product2/2, Product1/2  "Ls"
  Product1/1 -> Product3/1, Product5/1, σ/1  "σ"
  Constant/1 -> Add/2
  Product2/1 -> Add/1
  Math Function/1 -> Product2/1
  Product3/1 -> Product6/1, β/1  "β"
  Rr/1 -> Product4/1  "Rr"
  Product4/1 -> Product6/2, α/1  "α"
  Rs/1 -> Product5/2  "Rs"
  Product6/1 -> Add1/2  "γ"
  Product5/1 -> Add1/1
  Add1/1 -> γ/1

== system IM_Global_Control/(ab to dq transformation)/(ab to dq transformation)1 ==
  Isa : Inport
  Isb : Inport  Port=2
  ξ : Inport  Port=3
  Cos : Trigonometry  Operator=cos
  Cos1 : Trigonometry
  Product{,1..3} (4 alike) : Product
  Sin : Trigonometry
  Sin1 : Trigonometry  Operator=cos
  Subtract : Sum
  Subtract1 : Sum  Inputs=-+
  Isd : Outport
  Isq : Outport  Port=2
  wires:
  Subtract1/1 -> Isq/1  "Isb"
  Subtract/1 -> Isd/1  "Isa"
  ξ/1 -> Sin1/1, Cos1/1, Sin/1, Cos/1  "ξ"
  Cos/1 -> Product/1
  Sin/1 -> Product1/2
  Cos1/1 -> Product2/1
  Sin1/1 -> Product3/2
  Isa/1 -> Product2/2, Product/2
  Isb/1 -> Product3/1, Product1/1
  Product/1 -> Subtract/1
  Product1/1 -> Subtract/2
  Product2/1 -> Subtract1/1
  Product3/1 -> Subtract1/2

== system IM_Global_Control/(ab to dq transformation)/(dq to ab transformation)1 ==
  Ψra : Inport
  Ψrb : Inport  Port=2
  ξ : Inport  Port=3
  Cos : Trigonometry  Operator=cos
  Cos1 : Trigonometry
  Product{,1..3} (4 alike) : Product
  Sin : Trigonometry
  Sin1 : Trigonometry  Operator=cos
  Subtract : Sum
  Subtract1 : Sum  Inputs=-+
  Ψsd : Outport
  Ψsq : Outport  Port=2
  wires:
  Subtract1/1 -> Ψsq/1
  Subtract/1 -> Ψsd/1
  ξ/1 -> Sin1/1, Cos1/1, Sin/1, Cos/1  "ξ"
  Cos/1 -> Product/1
  Sin/1 -> Product1/2
  Cos1/1 -> Product2/1
  Sin1/1 -> Product3/2
  Ψra/1 -> Product2/2, Product/2
  Ψrb/1 -> Product3/1, Product1/1
  Product/1 -> Subtract/1
  Product1/1 -> Subtract/2
  Product2/1 -> Subtract1/1
  Product3/1 -> Subtract1/2

== system IM_Global_Control/(ab to dq transformation)/angle ==
  Isq : Inport
  ω : Inport  Port=2
  Ψ* : Inport  Port=3
  α : Inport  Port=4
  ηq : Inport  Port=5
  M : Inport  Port=6
  Add : Sum  Inputs=++-
  Discrete-Time Integrator : DiscreteIntegrator  SampleTime=-1  ICPrevOutput=DiscIntNeverNeededParam  ICPrevScaledInput=DiscIntNeverNeededParam
  Product : Product  Inputs=***/
  Product1 : Product  Inputs=*/
  ω0 : Outport
  ξ0 : Outport  Port=2
  wires:
  Ψ*/1 -> Product/4, Product1/2
  M/1 -> Product/3
  ω/1 -> Add/2
  α/1 -> Product/2
  Product/1 -> Add/1
  Discrete-Time Integrator/1 -> ξ0/1
  Add/1 -> ω0/1, Discrete-Time Integrator/1
  Product1/1 -> Add/3
  ηq/1 -> Product1/1
  Isq/1 -> Product/1

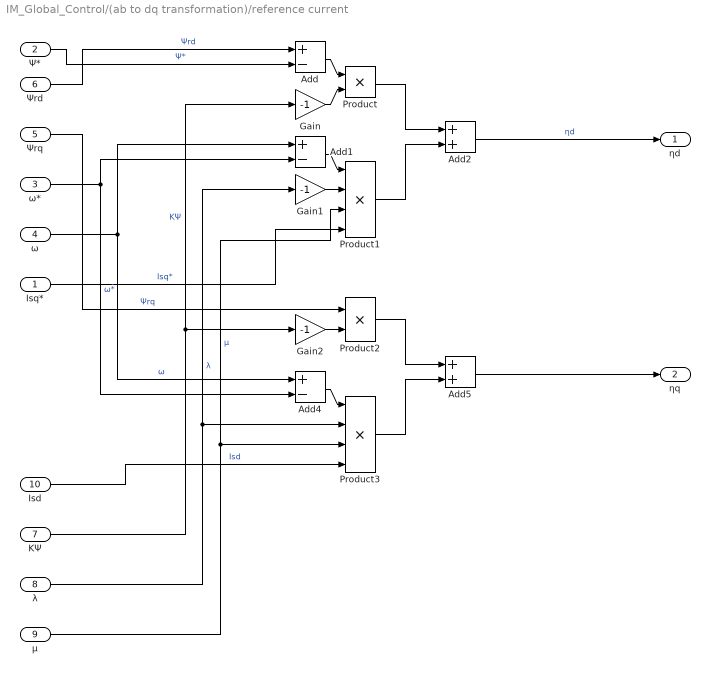
== system IM_Global_Control/(ab to dq transformation)/reference current ==
  Isq* : Inport
  Ψ* : Inport  Port=2
  ω* : Inport  Port=3
  ω : Inport  Port=4
  Ψrq : Inport  Port=5
  Ψrd : Inport  Port=6
  KΨ : Inport  Port=7
  λ : Inport  Port=8
  µ : Inport  Port=9
  Isd : Inport  Port=10
  Add : Sum  Inputs=+-
  Add1 : Sum  Inputs=+-
  Add2 : Sum
  Add4 : Sum  Inputs=+-
  Add5 : Sum
  Gain : Gain  Gain=-1
  Gain1 : Gain  Gain=-1
  Gain2 : Gain  Gain=-1
  Product : Product
  Product1 : Product  Inputs=4
  Product2 : Product
  Product3 : Product  Inputs=4
  ηd : Outport
  ηq : Outport  Port=2
  wires:
  Ψrd/1 -> Add/1  "Ψrd"
  Ψ*/1 -> Add/2  "Ψ*"
  Add/1 -> Product/1
  Gain/1 -> Product/2
  KΨ/1 -> Gain2/1, Gain/1  "KΨ"
  Add1/1 -> Product1/1
  Gain1/1 -> Product1/2
  ω/1 -> Add4/1, Add1/1  "ω"
  ω*/1 -> Add4/2, Add1/2  "ω*"
  λ/1 -> Gain1/1, Product3/2  "λ"
  µ/1 -> Product3/3, Product1/3  "µ"
  Product/1 -> Add2/1
  Product1/1 -> Add2/2
  Add2/1 -> ηd/1  "ηd"
  Add4/1 -> Product3/1
  Product3/1 -> Add5/2
  Product2/1 -> Add5/1
  Gain2/1 -> Product2/2
  Ψrq/1 -> Product2/1  "Ψrq"
  Isd/1 -> Product3/4  "Isd"
  Add5/1 -> ηq/1
  Isq*/1 -> Product1/4  "Isq*"

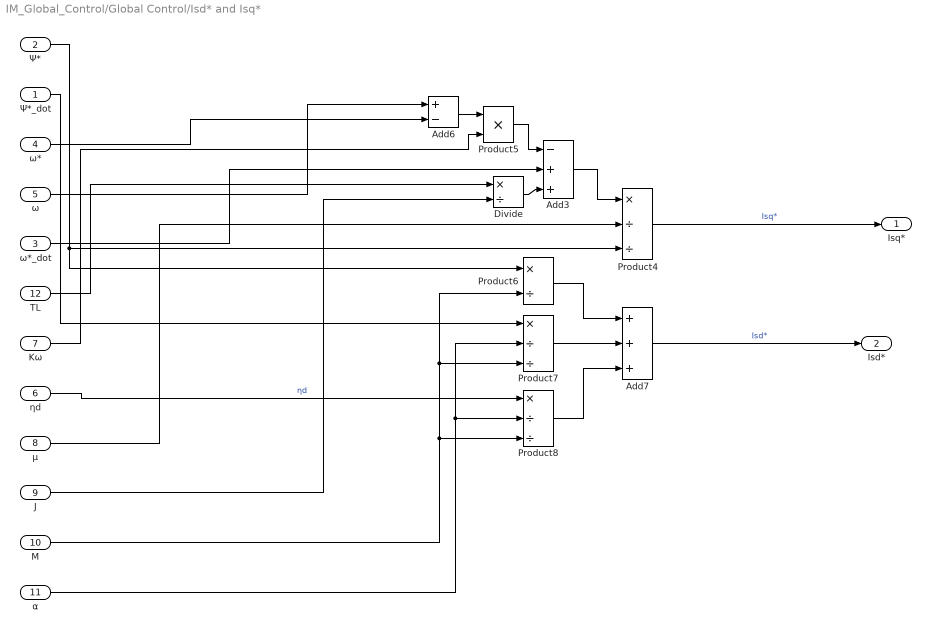
== system IM_Global_Control/Global Control/Isd* and Isq* ==
  Ψ*_dot : Inport
  Ψ* : Inport  Port=2
  ω*_dot : Inport  Port=3
  ω* : Inport  Port=4
  ω : Inport  Port=5
  ηd : Inport  Port=6
  Kω : Inport  Port=7
  µ : Inport  Port=8
  J : Inport  Port=9
  M : Inport  Port=10
  α : Inport  Port=11
  TL : Inport  Port=12
  Add3 : Sum  Inputs=-++
  Add6 : Sum  Inputs=+-
  Add7 : Sum  Inputs=+++
  Divide : Product  Inputs=*/
  Product4 : Product  Inputs=*//
  Product5 : Product
  Product6 : Product  Inputs=*/
  Product7 : Product  Inputs=*//
  Product8 : Product  Inputs=*//
  Isq* : Outport
  Isd* : Outport  Port=2
  wires:
  Kω/1 -> Product5/2
  M/1 -> Product6/2, Product7/3, Product8/3
  Ψ*/1 -> Product4/3, Product6/1
  µ/1 -> Product4/2
  ηd/1 -> Product8/1  "ηd"
  Divide/1 -> Add3/3
  ω*_dot/1 -> Add3/2
  ω*/1 -> Add6/2
  α/1 -> Product7/2, Product8/2
  Product8/1 -> Add7/3
  J/1 -> Divide/2
  ω/1 -> Add6/1
  Add6/1 -> Product5/1
  Product4/1 -> Isq*/1  "Isq*"
  Add3/1 -> Product4/1
  Ψ*_dot/1 -> Product7/1
  Product5/1 -> Add3/1
  Product6/1 -> Add7/1
  Product7/1 -> Add7/2
  Add7/1 -> Isd*/1  "Isd*"
  TL/1 -> Divide/1

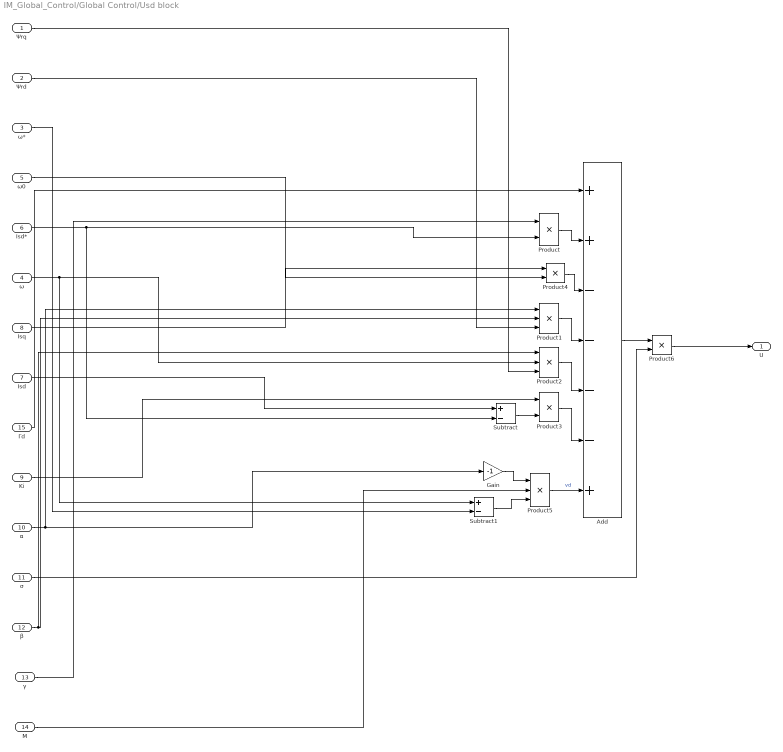
== system IM_Global_Control/Global Control/Usd block ==
  Ψrq : Inport
  Ψrd : Inport  Port=2
  ω* : Inport  Port=3
  ω : Inport  Port=4
  ω0 : Inport  Port=5
  Isd* : Inport  Port=6
  Isd : Inport  Port=7
  Isq : Inport  Port=8
  Ki : Inport  Port=9
  α : Inport  Port=10
  σ : Inport  Port=11
  β : Inport  Port=12
  γ : Inport  Port=13
  M : Inport  Port=14
  Γd : Inport  Port=15
  Add : Sum  Inputs=++----+
  Gain : Gain  Gain=-1
  Product{,3..4,6} (4 alike) : Product
  Product1 : Product  Inputs=3
  Product2 : Product  Inputs=3
  Product5 : Product  Inputs=3
  Subtract : Sum  Inputs=+-
  Subtract1 : Sum  Inputs=+-
  U : Outport
  wires:
  ω/1 -> Subtract1/1, Product2/2
  Product6/1 -> U/1
  Ψrd/1 -> Product1/3
  Product1/1 -> Add/4
  β/1 -> Product1/2, Product2/1
  Gain/1 -> Product5/1
  Add/1 -> Product6/1
  Product2/1 -> Add/5
  Product3/1 -> Add/6
  Subtract/1 -> Product3/2
  γ/1 -> Product/1
  α/1 -> Product1/1, Gain/1
  M/1 -> Product5/2
  Isd*/1 -> Subtract/2, Product/2
  ω0/1 -> Product4/2
  Product4/1 -> Add/3
  Product5/1 -> Add/7  "vd"
  Product/1 -> Add/2
  Subtract1/1 -> Product5/3
  Ki/1 -> Product3/1
  Isd/1 -> Subtract/1
  σ/1 -> Product6/2
  Ψrq/1 -> Product2/3
  Isq/1 -> Product4/1
  Γd/1 -> Add/1
  ω*/1 -> Subtract1/2

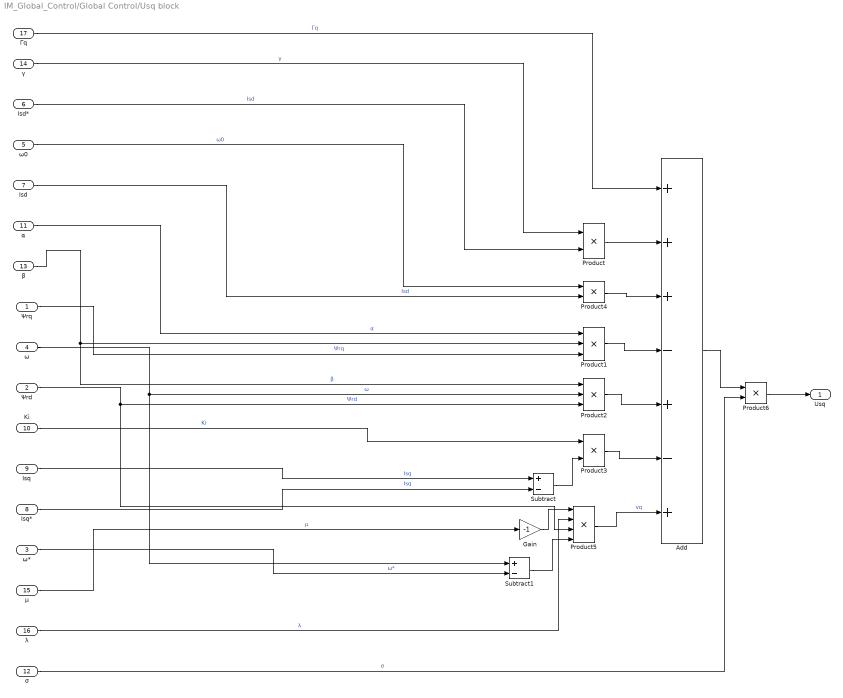
== system IM_Global_Control/Global Control/Usq block ==
  Ψrq : Inport
  Ψrd : Inport  Port=2
  ω* : Inport  Port=3
  ω : Inport  Port=4
  ω0 : Inport  Port=5
  Isd* : Inport  Port=6
  Isd : Inport  Port=7
  Isq* : Inport  Port=8
  Isq : Inport  Port=9
  Ki : Inport  Port=10
  α : Inport  Port=11
  σ : Inport  Port=12
  β : Inport  Port=13
  γ : Inport  Port=14
  µ : Inport  Port=15
  λ : Inport  Port=16
  Γq : Inport  Port=17
  Add : Sum  Inputs=+++-+-+
  Gain : Gain  Gain=-1
  Product{,3..4,6} (4 alike) : Product
  Product1 : Product  Inputs=3
  Product2 : Product  Inputs=3
  Product5 : Product  Inputs=4
  Subtract : Sum  Inputs=+-
  Subtract1 : Sum  Inputs=+-
  Usq : Outport
  wires:
  Product6/1 -> Usq/1
  Product1/1 -> Add/4
  β/1 -> Product1/2, Product2/1  "β"
  Gain/1 -> Product5/1
  Add/1 -> Product6/1
  Product2/1 -> Add/5
  Product3/1 -> Add/6
  Subtract/1 -> Product3/2
  α/1 -> Product1/1  "α"
  Product4/1 -> Add/3
  Product/1 -> Add/2
  Γq/1 -> Add/1  "Γq"
  γ/1 -> Product/1  "γ"
  Isd*/1 -> Product/2  "Isd"
  ω0/1 -> Product4/1  "ω0"
  Isd/1 -> Product4/2  "Isd"
  Ψrq/1 -> Product1/3  "Ψrq"
  ω/1 -> Subtract1/1, Product2/2  "ω"
  Ψrd/1 -> Product5/3, Product2/3  "Ψrd"
  Ki/1 -> Product3/1  "Ki"
  Isq/1 -> Subtract/1  "Isq"
  Isq*/1 -> Subtract/2  "Isq"
  ω*/1 -> Subtract1/2  "ω*"
  µ/1 -> Gain/1  "µ"
  λ/1 -> Product5/2  "λ"
  Subtract1/1 -> Product5/4
  Product5/1 -> Add/7  "vq"
  σ/1 -> Product6/2  "σ"

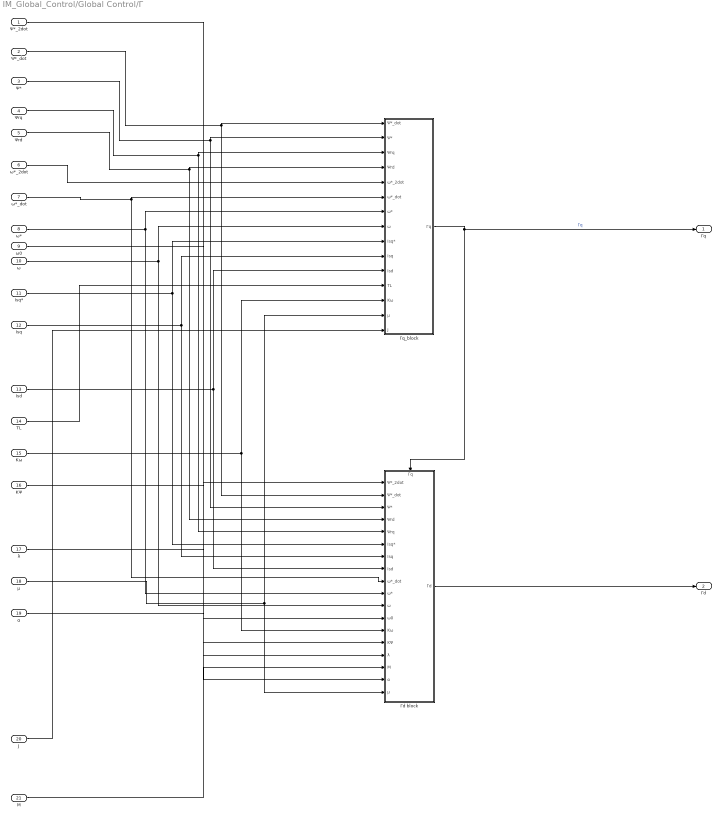
== system IM_Global_Control/Global Control/Γ ==
  Ψ*_2dot : Inport
  Ψ*_dot : Inport  Port=2
  Ψ* : Inport  Port=3
  Ψrq : Inport  Port=4
  Ψrd : Inport  Port=5
  ω*_2dot : Inport  Port=6
  ω*_dot : Inport  Port=7
  ω* : Inport  Port=8
  ω0 : Inport  Port=9
  ω : Inport  Port=10
  Isq* : Inport  Port=11
  Isq : Inport  Port=12
  Isd : Inport  Port=13
  TL : Inport  Port=14
  Kω : Inport  Port=15
  KΨ : Inport  Port=16
  λ : Inport  Port=17
  µ : Inport  Port=18
  α : Inport  Port=19
  J : Inport  Port=20
  M : Inport  Port=21
  Γd block : Subsystem
      settings: PortSchema="{\"entries\":[{\"content\":{\"sides\":[{\"content\":{\"connectorIds\":[\"In1\",\"In2\",\"In3\",\"In4\",\"In5\",\"In6\",\"In7\",\"In8\",\"In9\",\"In10\",\"In11\",\"In12\",\"In13\",\"In14\",\"In15\",\"In16\",\"In17\",\"In18\"]},\"type\":\"ConnectorPlacement.EquallySpacedRectSide\",\"uuid\":\"6c103e2d-eef5-457d-ab16-617f51de2bb6\"},{\"content\":{\"connectorIds\":[\"Out1\"],\"side\":\"RIGHT\"},\"type\":\"ConnectorPlacement.EquallySpacedRectSide\",\"uuid\":\"d0060888-85cb-49dc-96d4-360cb55f979d\"},{\"content\":{\"connectorIds\":[\"In19\"],\"side\":\"TOP\"},\"type\":\"ConnectorPlacement.EquallySpacedRectSide\",\"uuid\":\"c309ca79-9ccc-4e7a-81b6-dbd7fe2c6fbb\"}]},\"type\":\"ConnectorPlacement.EquallySpacedConnector\",\"uuid\":\"e9330f3c-ebb7-4d09-a354-84c6ad186824\"}],\"packageUris\":[\"http://schema.mathworks.com/mf0/Connector/R2020b\"],\"version\":\"1.0\"}"
  Γq_block : Subsystem
  Γq : Outport
  Γd : Outport  Port=2
  wires:
  Ψ*_dot/1 -> Γd block/2(Ψ*_dot), Γq_block/1(Ψ*_dot)
  Ψrq/1 -> Γd block/5(Ψrq), Γq_block/3(Ψrq)
  Γd block/1(Γd) -> Γd/1
  Ψrd/1 -> Γd block/4(Ψrd), Γq_block/4(Ψrd)
  ω/1 -> Γd block/11(ω), Γq_block/8(ω)
  Γq_block/1(Γq) -> Γq/1, Γd block/19(Γq)  "Γq"
  Isd/1 -> Γd block/8(Isd), Γq_block/11(Isd)
  Isq*/1 -> Γd block/6(Isq*), Γq_block/9(Isq*)
  ω*/1 -> Γd block/10(ω*), Γq_block/7(ω*)
  Kω/1 -> Γd block/13(Kω), Γq_block/13(Kω)
  Isq/1 -> Γd block/7(Isq), Γq_block/10(Isq)
  KΨ/1 -> Γd block/14(KΨ)
  α/1 -> Γd block/17(α)
  λ/1 -> Γd block/15(λ)
  µ/1 -> Γq_block/14(µ), Γd block/18(µ)
  ω*_dot/1 -> Γq_block/6(ω*_dot), Γd block/9(ω*_dot)
  Ψ*/1 -> Γd block/3(Ψ*), Γq_block/2(Ψ*)
  M/1 -> Γd block/16(M)
  Ψ*_2dot/1 -> Γd block/1(Ψ*_2dot)
  J/1 -> Γq_block/15(J)
  ω0/1 -> Γd block/12(ω0)
  ω*_2dot/1 -> Γq_block/5(ω*_2dot)
  TL/1 -> Γq_block/12(TL)

== system IM_Global_Control/Observers/modulus ==
  1 : Inport
  In2 : Inport  Port=2
  Add : Sum
  Math Function : Math  Operator=square  SaturateOnIntegerOverflow=on
  Math Function1 : Math  Operator=square  SaturateOnIntegerOverflow=on
  Sqrt : Sqrt  SaturateOnIntegerOverflow=on
  Output : Outport
  wires:
  Add/1 -> Sqrt/1
  In2/1 -> Math Function1/1
  1/1 -> Math Function/1
  Math Function1/1 -> Add/2
  Math Function/1 -> Add/1
  Sqrt/1 -> Output/1

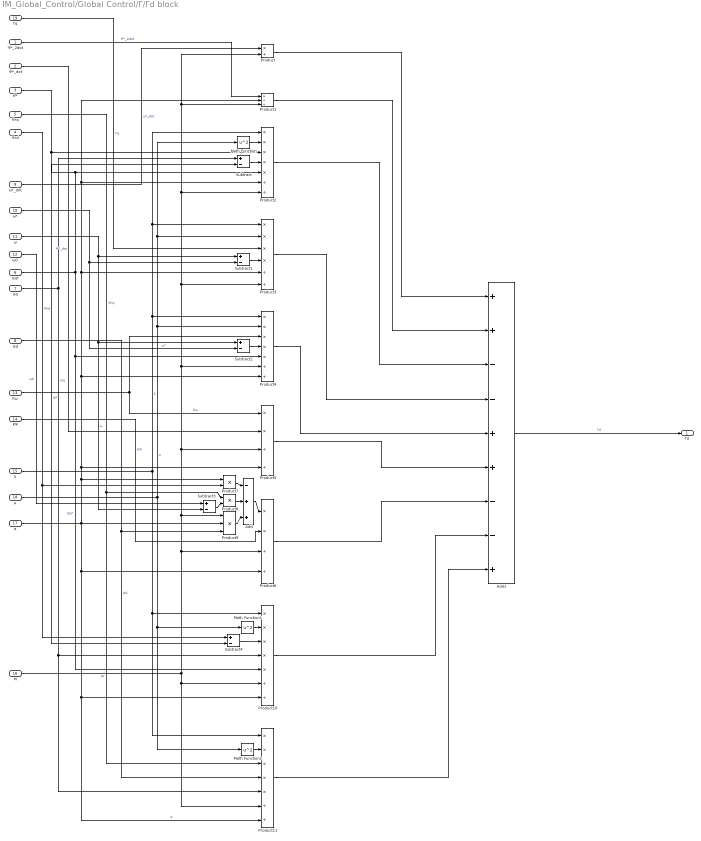
== system IM_Global_Control/Global Control/Γ/Γd block ==
  Ψ*_2dot : Inport
  Ψ*_dot : Inport  Port=2
  Ψ* : Inport  Port=3
  Ψrd : Inport  Port=4
  Ψrq : Inport  Port=5
  Isq* : Inport  Port=6
  Isq : Inport  Port=7
  Isd : Inport  Port=8
  ω*_dot : Inport  Port=9
  ω* : Inport  Port=10
  ω : Inport  Port=11
  ω0 : Inport  Port=12
  Kω : Inport  Port=13
  KΨ : Inport  Port=14
  λ : Inport  Port=15
  M : Inport  Port=16
  α : Inport  Port=17
  µ : Inport  Port=18
  Γq : Inport  Port=19
  Add : Sum  Inputs=-++
  Add1 : Sum  Inputs=++--++--+
  Math Function : Math  Operator=square  SaturateOnIntegerOverflow=on
  Math Function1 : Math  Operator=square  SaturateOnIntegerOverflow=on
  Math Function2 : Math  Operator=square  SaturateOnIntegerOverflow=on
  Product : Product  Inputs=*/
  Product1 : Product  Inputs=*//
  Product{2,4,10..11} (4 alike) : Product  Inputs=*****//
  Product3 : Product  Inputs=****//
  Product5 : Product  Inputs=**//
  Product6 : Product  Inputs=**//
  Product7 : Product
  Product8 : Product
  Product9 : Product  Inputs=3
  Subtract{,1..4} (5 alike) : Sum  Inputs=+-
  Γd : Outport
  wires:
  ω*_dot/1 -> Product/1  "ω*_dot"
  M/1 -> Product11/6, Product10/6, Product9/1, Product5/3, Product4/6, Product3/6, Product2/7, Product1/3, Product/2, Product6/3  "M"
  Ψ*_2dot/1 -> Product1/1  "Ψ*_2dot"
  α/1 -> Product11/7, Product10/7, Product6/4, Product9/2, Product7/1, Product4/7, Product1/2, Product2/6, Product3/5, Product5/4  "α"
  λ/1 -> Product11/1, Product10/1, Product4/1, Product3/1, Product2/1  "λ"
  Math Function/1 -> Product2/2
  µ/1 -> Math Function2/1, Math Function1/1, Math Function/1, Product3/2, Product4/2  "µ"
  Ψ*/1 -> Product2/3, Subtract4/2  "Ψ*"
  Subtract/1 -> Product2/4
  Isq*/1 -> Subtract/2, Product2/5, Product10/5, Product4/5  "Isq*"
  Isq/1 -> Product11/5, Product10/4, Subtract/1  "Isq"
  Γq/1 -> Product3/3  "Γq"
  Subtract1/1 -> Product3/4
  ω/1 -> Subtract3/2, Subtract2/1, Subtract1/1  "ω"
  ω*/1 -> Subtract2/2, Subtract1/2  "ω*"
  Subtract2/1 -> Product4/4
  Kω/1 -> Product5/1, Product4/3  "Kω"
  Ψ*_dot/1 -> Product5/2  "Ψ*_dot"
  KΨ/1 -> Product6/2  "KΨ"
  Add/1 -> Product6/1
  Product7/1 -> Add/1
  Ψrd/1 -> Subtract4/1, Product7/2  "Ψrd"
  Product8/1 -> Add/2
  Subtract3/1 -> Product8/2
  Ψrq/1 -> Product11/3, Product8/1  "Ψrq"
  ω0/1 -> Subtract3/1  "ω0"
  Product9/1 -> Add/3
  Isd/1 -> Product11/4, Product9/3  "Isd"
  Math Function1/1 -> Product10/2
  Subtract4/1 -> Product10/3
  Math Function2/1 -> Product11/2
  Product/1 -> Add1/1
  Product1/1 -> Add1/2
  Product2/1 -> Add1/3
  Add1/1 -> Γd/1  "Γd"
  Product3/1 -> Add1/4
  Product4/1 -> Add1/5
  Product5/1 -> Add1/6
  Product6/1 -> Add1/7
  Product10/1 -> Add1/8
  Product11/1 -> Add1/9

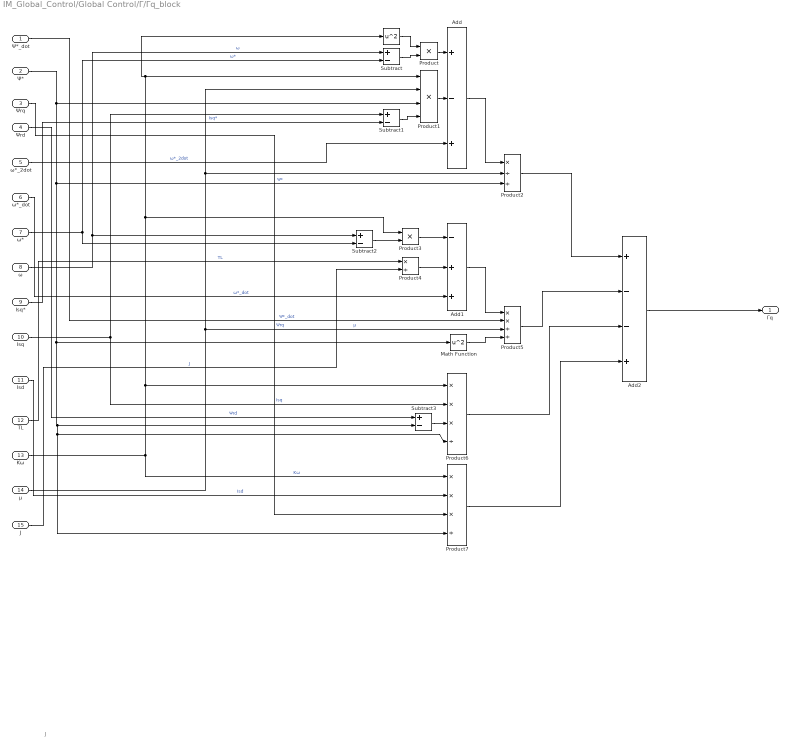
== system IM_Global_Control/Global Control/Γ/Γq_block ==
  note: J
  Ψ*_dot : Inport
  Ψ* : Inport  Port=2
  Ψrq : Inport  Port=3
  Ψrd : Inport  Port=4
  ω*_2dot : Inport  Port=5
  ω*_dot : Inport  Port=6
  ω* : Inport  Port=7
  ω : Inport  Port=8
  Isq* : Inport  Port=9
  Isq : Inport  Port=10
  Isd : Inport  Port=11
  TL : Inport  Port=12
  Kω : Inport  Port=13
  µ : Inport  Port=14
  J : Inport  Port=15
  " " : Math  Operator=square  SaturateOnIntegerOverflow=on
  Add : Sum  Inputs=+-+
  Add1 : Sum  Inputs=-++
  Add2 : Sum  Inputs=+--+
  Math Function : Math  Operator=square  SaturateOnIntegerOverflow=on
  Product : Product
  Product1 : Product  Inputs=4
  Product2 : Product  Inputs=*//
  Product3 : Product
  Product4 : Product  Inputs=*/
  Product5 : Product  Inputs=**//
  Product6 : Product  Inputs=***/
  Product7 : Product  Inputs=***/
  Subtract{,1..3} (4 alike) : Sum  Inputs=+-
  Γq : Outport
  wires:
  Product7/1 -> Add2/4
  " "/1 -> Product/1
  Subtract2/1 -> Product3/2
  Ψ*/1 -> Product1/3, Product2/3, Subtract3/2, Product7/4, Product6/4, Math Function/1  "Ψ*"
  ω/1 -> Subtract2/1, Subtract/1  "ω"
  Ψrd/1 -> Subtract3/1  "Ψrd"
  Product1/1 -> Add/2
  Add1/1 -> Product5/1
  Product/1 -> Add/1
  µ/1 -> Product5/3, Product2/2, Product1/2  "µ"
  Subtract1/1 -> Product1/4
  ω*/1 -> Subtract2/2, Subtract/2  "ω*"
  Add2/1 -> Γq/1
  Kω/1 -> Product7/1, Product6/1, " "/1, Product1/1, Product3/1  "Kω"
  Product5/1 -> Add2/2
  Isq/1 -> Product6/2, Subtract1/1  "Isq"
  Product4/1 -> Add1/2
  Product6/1 -> Add2/3
  Subtract3/1 -> Product6/3
  Ψ*_dot/1 -> Product5/2  "Ψ*_dot"
  Isq*/1 -> Subtract1/2  "Isq*"
  Product2/1 -> Add2/1
  Ψrq/1 -> Product7/3  "Ψrq"
  Add/1 -> Product2/1
  Product3/1 -> Add1/1
  Subtract/1 -> Product/2
  Isd/1 -> Product7/2  "Isd"
  J/1 -> Product4/2  "J"
  Math Function/1 -> Product5/4
  TL/1 -> Product4/1  "TL"
  ω*_dot/1 -> Add1/3  "ω*_dot"
  ω*_2dot/1 -> Add/3  "ω*_2dot"
